simulink model "input_integrator"  (R2014b)
settings: Solver=ode3  SolverMode=SingleTasking  StartTime=0.0  StopTime=Tsim  FixedStep=Ts  RelTol=1e-3
InitFcn:
  | configIntegrator
values from neighbouring files (symbols this model uses):
  acc = -3    [integratorCaseTest.m]
  changeacc = -3    [integratorCaseTest.m]
  v_0 = 0    [integratorCaseTest.m]
  v_max = 25    [integratorCaseTest.m]
  v_min = -25    [integratorCaseTest.m]
settings Model: CovMetricSettings=dwe  CovHtmlReporting=off  covSaveCumulativeToWorkspaceVar=off  CovSaveSingleToWorkspaceVar=off  CovExternalEMLEnable=on  CovSFcnEnable=on  Creator=mnade  LastModifiedBy=nina
settings DataIOCC: LimitDataPoints=off  SaveFormat=StructureWithTime
settings DebuggingCC: SolverPrmCheckMsg=none  FrameProcessingCompatibilityMsg=error  SFUnexpectedBacktrackingDiag=error  SFNoUnconditionalDefaultTransitionDiag=error
settings HardwareCC: ProdBitPerPointer=64  ProdLargestAtomicFloat=Float  ProdIntDivRoundTo=Zero  ProdEndianess=LittleEndian  ProdHWDeviceType=Specified
settings ModelReferenceCC: PropagateSignalLabelsOutOfModel=on
settings GRTTargetCC: TargetLangStandard=C99 (ISO)  GeneratePreprocessorConditionals=Use local settings

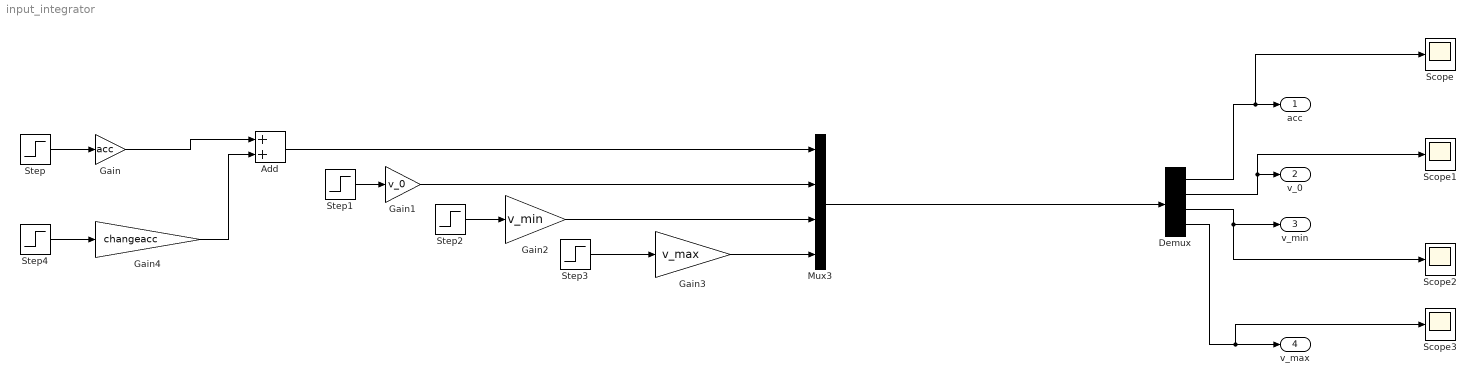
== system input_integrator ==
  Add : Sum
  Demux : Demux
  Gain : Gain  Gain=acc
  Gain1 : Gain  Gain=v_0
  Gain2 : Gain  Gain=v_min
  Gain3 : Gain  Gain=v_max
  Gain4 : Gain  Gain=changeacc
  Mux3 : Mux
  Scope{,1..3} (4 alike) : Scope
      Scope2 settings: SaveName=ScopeData2
      Scope3 settings: SaveName=ScopeData3
  Step{,1..3} (4 alike) : Step  Time=0  SampleTime=0
  Step4 : Step  Time=15  After=-2  SampleTime=0
  acc : Outport
  v_0 : Outport  Port=2
  v_min : Outport  Port=3
  v_max : Outport  Port=4
  wires:
  Demux/1 -> Scope/1, acc/1
  Demux/2 -> Scope1/1, v_0/1
  Demux/3 -> Scope2/1, v_min/1
  Demux/4 -> Scope3/1, v_max/1
  Gain3/1 -> Mux3/4
  Gain2/1 -> Mux3/3
  Gain1/1 -> Mux3/2
  Mux3/1 -> Demux/1
  Step/1 -> Gain/1
  Step1/1 -> Gain1/1
  Step2/1 -> Gain2/1
  Step3/1 -> Gain3/1
  Step4/1 -> Gain4/1
  Add/1 -> Mux3/1
  Gain/1 -> Add/1
  Gain4/1 -> Add/2
